simulink model "subsystems"  (R2024b)
settings: Solver=VariableStepAuto  StartTime=0.0  StopTime=10.0  RelTol=1e-3
libraries: simulink x1
settings Model: Creator=Ahmad  LastModifiedBy=Ahmad

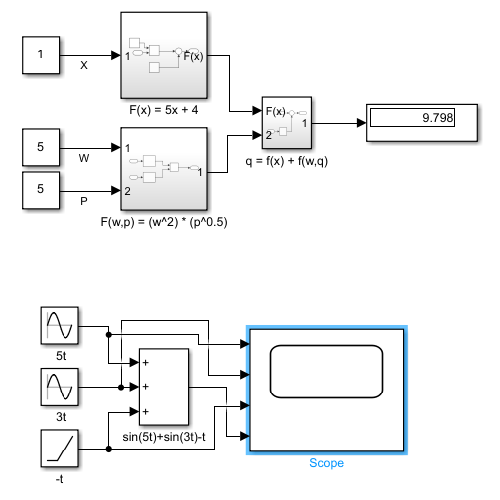
[thumbnail: Simulink's stored preview of the top-level diagram]
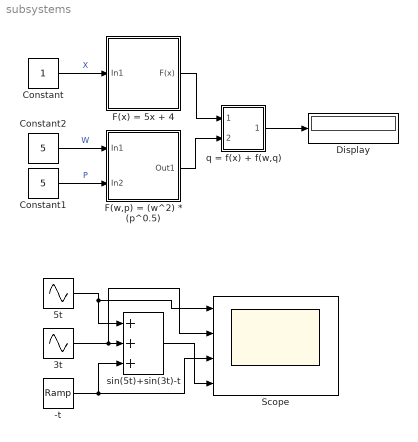
== system subsystems ==
  " 3t" : Sin  Frequency=3  SampleTime=0
  " 5t" : Sin  Frequency=5  SampleTime=0
  -t : simulink/Sources/Ramp  slope=-1  start=0  InitialOutput=0
  Constant : Constant
  Constant1 : Constant  Value=5
  Constant2 : Constant  Value=5
  Display : Display
  F(w,p) = (w^2) * (p^0.5) : Subsystem
  F(x) = 5x + 4 : Subsystem
  Scope : Scope  NumInputPorts=4
  q = f(x) + f(w,q) : Subsystem
  sin(5t)+sin(3t)-t : Sum  Inputs=+++
  wires:
  Constant/1 -> F(x) = 5x + 4/1(In1)  "X"
  Constant2/1 -> F(w,p) = (w^2) * (p^0.5)/1(In1)  "W"
  Constant1/1 -> F(w,p) = (w^2) * (p^0.5)/2(In2)  "P"
  F(w,p) = (w^2) * (p^0.5)/1(Out1) -> q = f(x) + f(w,q)/2(In2)
  F(x) = 5x + 4/1(F(x)) -> q = f(x) + f(w,q)/1(F(x))
  q = f(x) + f(w,q)/1(Out1) -> Display/1
  " 5t"/1 -> Scope/1, sin(5t)+sin(3t)-t/1
  " 3t"/1 -> Scope/2, sin(5t)+sin(3t)-t/2
  -t/1 -> Scope/3, sin(5t)+sin(3t)-t/3
  sin(5t)+sin(3t)-t/1 -> Scope/4

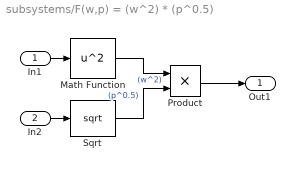
== system subsystems/F(w,p) = (w^2) * (p^0.5) ==
  In1 : Inport
  In2 : Inport  Port=2
  Math Function : Math  Operator=square
  Product : Product
  Sqrt : Sqrt
  Out1 : Outport
  wires:
  Math Function/1 -> Product/1  "(w^2)"
  In2/1 -> Sqrt/1
  Sqrt/1 -> Product/2  "(p^0.5)"
  Product/1 -> Out1/1
  In1/1 -> Math Function/1

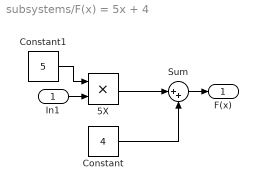
== system subsystems/F(x) = 5x + 4 ==
  In1 : Inport
  5X : Product
  Constant : Constant  Value=4
  Constant1 : Constant  Value=5
  Sum : Sum  Inputs=|++
  F(x) : Outport
  wires:
  Constant/1 -> Sum/2
  5X/1 -> Sum/1
  Sum/1 -> F(x)/1
  Constant1/1 -> 5X/1
  In1/1 -> 5X/2

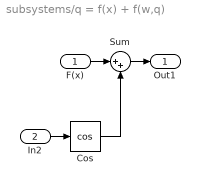
== system subsystems/q = f(x) + f(w,q) ==
  F(x) : Inport
  In2 : Inport  Port=2
  Cos : Trigonometry  Operator=cos
  Sum : Sum  Inputs=|++
  Out1 : Outport
  wires:
  Cos/1 -> Sum/2
  F(x)/1 -> Sum/1
  In2/1 -> Cos/1
  Sum/1 -> Out1/1
